simulink subsystem "led"  (R2024a)
settings: Solver=VariableStepAuto  StartTime=0.0  StopTime=10.0  RelTol=1e-3
libraries: arduinolib x4, simulink x1
settings Model: Creator=Usuario_UMA  LastModifiedBy=julia
settings RTWCC: GPUComputeCapability=3.5

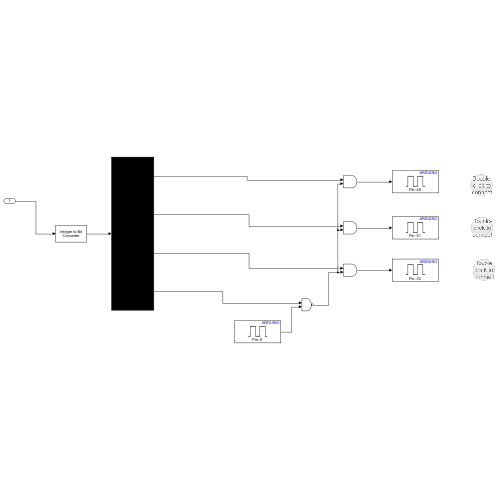
[thumbnail: Simulink's stored preview of the top-level diagram]
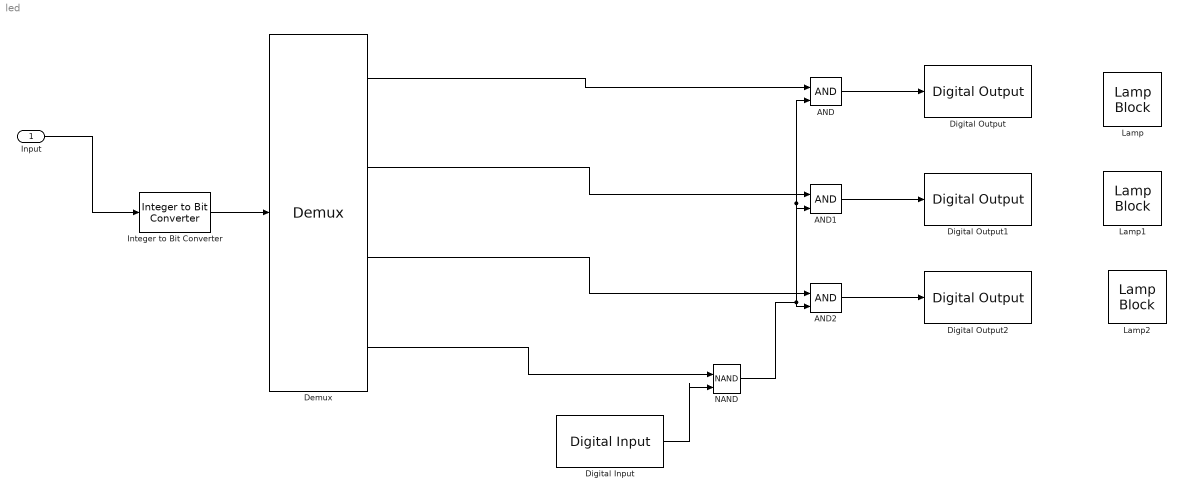
== system led ==
  Input : Inport
  AND : Logic  IconShape=distinctive  AllPortsSameDT=off  OutDataTypeStr=boolean
  AND1 : Logic  IconShape=distinctive  AllPortsSameDT=off  OutDataTypeStr=boolean
  AND2 : Logic  IconShape=distinctive  AllPortsSameDT=off  OutDataTypeStr=boolean
  Demux : Demux
  Digital Input : arduinolib/Digital Input  pinNumber=8  mode=Default  Direction=input  SampleTime=0.1  blockPlatform=arduino
  Digital Output : arduinolib/Digital Output  pinNumber=49  Direction=output  blockPlatform=arduino
  Digital Output1 : arduinolib/Digital Output  pinNumber=51  Direction=output  blockPlatform=arduino
  Digital Output2 : arduinolib/Digital Output  pinNumber=53  Direction=output  blockPlatform=arduino
  Integer to Bit Converter : simulink/Logic and Bit Operations/Integer to Bit Converter  nbits=4  signedInputValues=Unsigned  bitOrder=MSB first  outDtype=boolean
  Lamp : LampBlock  LabelPosition=Hide
  Lamp1 : LampBlock  LabelPosition=Hide
  Lamp2 : LampBlock  LabelPosition=Hide
  NAND : Logic  Operator=NAND  IconShape=distinctive  AllPortsSameDT=off  OutDataTypeStr=boolean
  wires:
  AND/1 -> Digital Output/1
  AND1/1 -> Digital Output1/1
  AND2/1 -> Digital Output2/1
  Integer to Bit Converter/1 -> Demux/1
  Digital Input/1 -> NAND/2
  Demux/1 -> AND/1
  Demux/2 -> AND1/1
  Demux/3 -> AND2/1
  Demux/4 -> NAND/1
  Input/1 -> Integer to Bit Converter/1
  NAND/1 -> AND/2, AND1/2, AND2/2
